simulink model "L0702"  (R2022b)
settings: Solver=FixedStepDiscrete  StartTime=0.0  StopTime=100  FixedStep=1  RelTol=1e-3
settings Model: Creator=Andrey  LastModifiedBy=Andrey

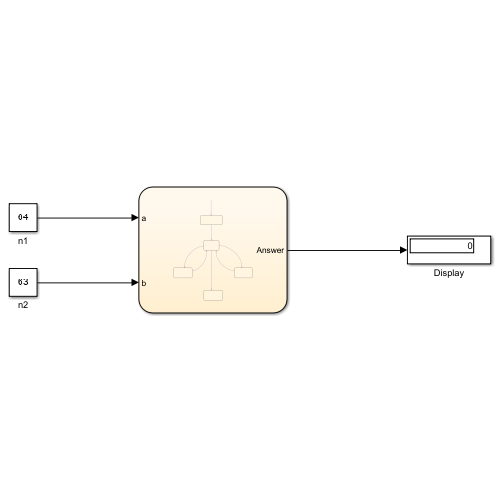
[thumbnail: Simulink's stored preview of the top-level diagram]
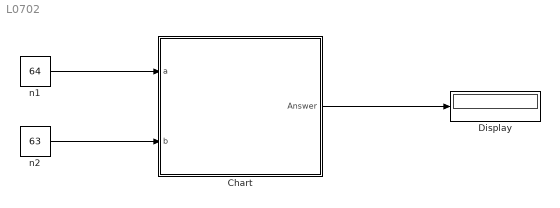
== system L0702 ==
  Chart : Stateflow chart  TreatAsAtomicUnit=on
  Display : Display
  n1 : Constant  Value=64
  n2 : Constant  Value=63
  wires:
  Chart/1(Answer) -> Display/1
  n2/1 -> Chart/2(b)
  n1/1 -> Chart/1(a)

== stateflow chart L0702/Chart ==
  state Entr
    entry: n1 = a; n2 = b;
  state Loop
  state Less
    entry: n2 = n2 - n1;
  state Greater
    entry: n1 = n1 - n2;
  state Equal
    entry: Answer = n1;
  (default) -> Entr
  Entr -> Loop
  Loop -> Greater [order 3] : [n1 > n2]
  Loop -> Less [order 2] : [n2 > n1]
  Less -> Loop
  Loop -> Equal [order 1] : [n1 == n2]
  Greater -> Loop
  data: Answer output; a input; b input; n1 local; n2 local
